simulink model "pokus1"  (R2014a)
settings: Solver=ode45  StartTime=0.0  StopTime=10.0  RelTol=1e-3
libraries: legonxtlib x4
settings Model: ExtModeTrigDuration=2  Creator=David  LastModifiedBy=David
settings OptimizationCC: OptimizeModelRefInitCode=on  LifeSpan=1
settings DebuggingCC: UnderspecifiedInitializationDetection=Classic  StrictBusMsg=Warning
settings HardwareCC: ProdBitPerInt=16  ProdBitPerPointer=8  ProdIntDivRoundTo=Zero  ProdEndianess=LittleEndian  ProdWordSize=8  ProdHWDeviceType=Atmel->AVR
settings RTWCC: SystemTargetFile=realtime.tlc  GenerateMakefile=off  TemplateMakefile=realtime.tmf  Description=Run on Target Hardware  RTWVerbose=off  ProcessScript=realtime_make_rtw_hook
settings CodeAppCC: IgnoreCustomStorageClasses=off
settings STFCustomTargetCC: TargetLibSuffix=.a  GenerateSampleERTMain=on  ConcurrentExecutionCompliant=off  GeneratePreprocessorConditionals=Use local settings  CombineOutputUpdateFcns=on  ERTCustomFileBanners=on  SupportContinuousTime=off  SupportNonInlinedSFcns=off  MATLABClassNameForMDSCustomization=Simulink.SoftwareTarget.ERTCustomization  GRTInterface=off  SystemTargetFile=realtime.tlc
settings ERTTargetCC: ERTCustomFileTemplate=realtime_file_process.tlc

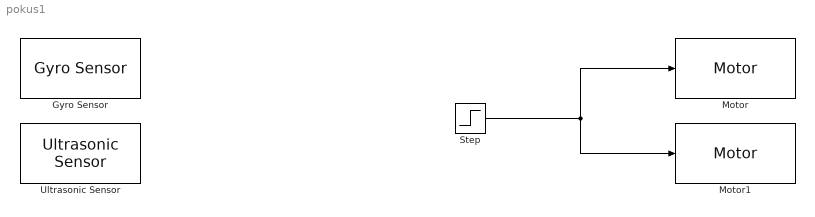
== system pokus1 ==
  Gyro Sensor : legonxtlib/Gyro Sensor  portNumber=4  outputMode=Rotation rate (-360 - 360)  offset=600  sampleTime=0.1
  Motor : legonxtlib/Motor  sportNumber=B  sstopAction=Brake
  Motor1 : legonxtlib/Motor  sportNumber=C  sstopAction=Brake
  Step : Step  SampleTime=0
  Ultrasonic Sensor : legonxtlib/Ultrasonic Sensor  PortNumber=2  sampleTime=0.1
  wires:
  Step/1 -> Motor/1, Motor1/1
